simulink model "leader_qbot2"  (Simulink 8.3)
settings: Solver=ode1  StartTime=0.0  StopTime=inf  FixedStep=0.002  RelTol=1e-3
undefined symbols (not defined in the file or in its folder): HIL
libraries: quarc_library x13, simulink x1
settings Model: Creator=glai  LastModifiedBy=user  SimulationMode=external  ExtModeTrigDuration=5000
settings SolverCC: PositivePriorityOrder=on
settings DataIOCC: SignalLoggingSaveFormat=Dataset
settings OptimizationCC: ExpressionDepthLimit=2147483647
settings RTWCC: SystemTargetFile=quarc_linux_duovero.tlc  TemplateMakefile=quarc_linux_duovero_tmf  Description=QUARC Linux DuoVero Target (QBall 2, QBot 2)  ProcessScript=quarc_linux_duovero_make_rtw_hook
settings STFCustomTargetCC: TargetLibSuffix=.a  TargetPreCompLibLocation=C:\PROGRA~3\QUARC\lib\2014a\LINUX_~3\release  CodeReplacementLibrary=C89/C90 (ANSI)  ConcurrentExecutionCompliant=on  GeneratePreprocessorConditionals=Disable all  CombineOutputUpdateFcns=on  CPPClassGenCompliant=on  GRTInterface=off  SystemTargetFile=quarc_linux_duovero.tlc
settings GRTTargetCC: TargetLibSuffix=.a  TargetPreCompLibLocation=C:\PROGRA~3\QUARC\lib\2014a\LINUX_~3\release  CodeReplacementLibrary=C89/C90 (ANSI)  ParMdlRefBuildCompliant=off  CompOptLevelCompliant=off  CombineOutputUpdateFcns=on  MatFileLogging=off  GRTInterface=off  ExtMode=on  ExtModeMexFile=quarc_comm  ExtModeMexArgs='-w -d /tmp -uri %u', 'tcpip://192.168.2.47:17001?nagle=no,keep_alive=1'

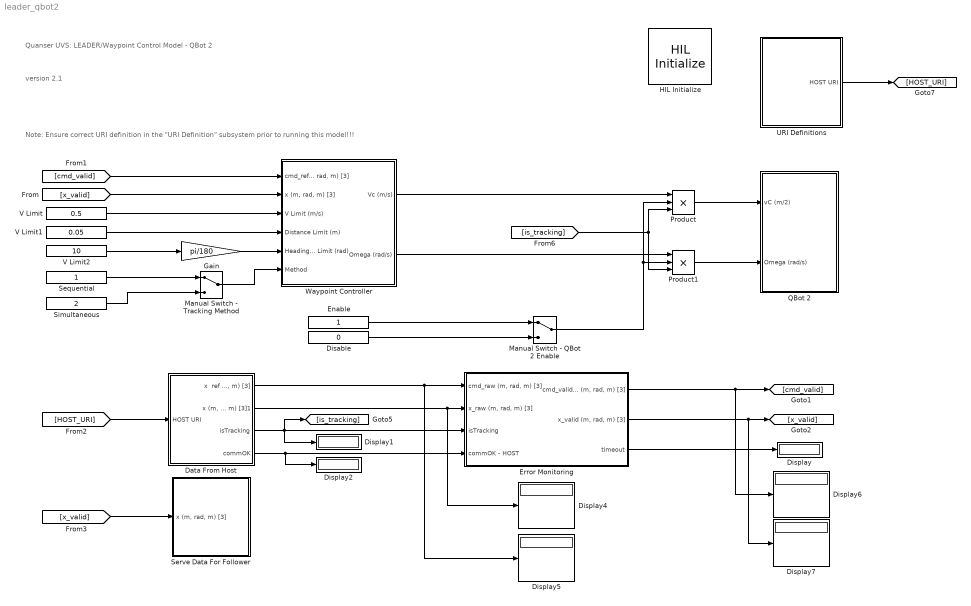
== system leader_qbot2 ==
  note: version 2.1
  note: Note: Ensure correct URI definition in the "URI Definition" subsystem prior to running this model!!!
  note: Quanser UVS: LEADER/Waypoint Control Model - QBot 2
  Data From Host : Subsystem
  Disable : Constant  Value=0
  Display{,1..2,4..7} (7 alike) : Display
      settings: Decimation=100
  Enable : Constant
  Error Monitoring : Subsystem
  Gain : Gain  Gain=pi/180
  HIL Initialize : quarc_library/Data Acquisition/Generic/Configuration/HIL Initialize  Priority=-99  object_name=HIL-1  board_type=qbot2  board_number=0  board_options=enc0_dir=0;enc0_filter=1;enc0_a=0;enc0_b=0;enc0_z=1;enc0_reload=0;enc1_dir=0;enc1_filter=1;enc1_a=0;enc1_b=0;enc1_z=1;enc1_reload=0;pwm0_immediate=0;pwm1_immediate=0;pwm2_immediate=0;pwm3_immediate=0;  exclusive=off  active=off  hardware_clocks=[]  clock_modes=[]  initial_clock_frequencies=[]  set_clock_params_at_start=off  set_clock_params_at_switch_in=off  set_clock_frequencies_at_start=off  set_clock_frequencies_at_switch_in=off  analog_input_channels=[0:9]  analog_input_maximums=[5 5 5 5 16.5 3.3 3.3 3.3 3.3]  analog_input_minimums=[0 0 0 0 0 0 0 0 0]  set_analog_input_params_at_start=off  set_analog_input_params_at_switch_in=off  analog_output_channels=[]  analog_output_maximums=[]  analog_output_minimums=[]  initial_analog_outputs=[]  final_analog_outputs=[]  watchdog_analog_outputs=[]  set_analog_output_params_at_start=off  set_analog_output_params_at_switch_in=off  set_analog_outputs_at_start=off  set_analog_outputs_at_switch_in=off  set_analog_outputs_at_terminate=off  set_analog_outputs_at_switch_out=off  set_analog_outputs_on_watchdog=off  digital_input_channels=[]  digital_output_channels=[]  digital_output_configuration=[]  initial_digital_outputs=[0]  final_digital_outputs=[0]  watchdog_digital_outputs=[0]  set_digital_output_params_at_start=off  set_digital_output_params_at_switch_in=off  set_digital_outputs_at_start=on  set_digital_outputs_at_switch_in=off  set_digital_outputs_at_terminate=on  set_digital_outputs_at_switch_out=off  set_digital_outputs_on_watchdog=on  encoder_channels=[0:3]  quadrature=[4]  encoder_filter_frequency=[]  initial_encoder_counts=[0]  set_encoder_params_at_start=on  set_encoder_params_at_switch_in=off  set_encoder_counts_at_start=on  set_encoder_counts_at_switch_in=off  pwm_channels=[0:3]  pwm_modes=[0]  pwm_frequency=[20e6/1024]  pwm_configuration=[0]  pwm_alignment=[0]  pwm_polarity=[1]  pwm_leading_deadband=[0]  pwm_trailing_deadband=[0]  initial_pwm_outputs=[0]  final_pwm_outputs=[0]  watchdog_pwm_outputs=[0]  set_pwm_params_at_start=on  set_pwm_params_at_switch_in=off  set_pwm_outputs_at_start=on  set_pwm_outputs_at_switch_in=off  set_pwm_outputs_at_terminate=on  set_pwm_outputs_at_switch_out=off  set_pwm_outputs_on_watchdog=on  other_output_channels=[2000:2001 14000 16000]  initial_other_outputs=[0 0 0 7]  final_other_outputs=[0 0 0 7]  watchdog_other_outputs=[]  set_other_outputs_at_start=on  set_other_outputs_at_switch_in=off  set_other_outputs_at_terminate=on  set_other_outputs_at_switch_out=off  set_other_outputs_on_watchdog=off
  Manual Switch - QBot 2 Enable : ManualSwitch
  Manual Switch - Tracking Method : ManualSwitch
  Product : Product  Inputs=3  RndMeth=Zero
  Product1 : Product  Inputs=3  RndMeth=Zero
  QBot 2 : Subsystem
  Sequential : Constant
  Serve Data For Follower : Subsystem
  Simultaneous : Constant  Value=2
  URI Definitions : Subsystem
  V Limit : Constant  Value=0.5
  V Limit1 : Constant  Value=0.05
  V Limit2 : Constant  Value=10
  Waypoint Controller : Subsystem
  wires:
  URI Definitions/1(HOST URI) -> [HOST_URI]
  [HOST_URI] -> Data From Host/1(HOST URI)
  Data From Host/3(isTracking) -> Error Monitoring/3(isTracking), Display1/1, [is_tracking]
  Data From Host/4(commOK) -> Display2/1, Error Monitoring/4(commOK - HOST)
  Error Monitoring/2("x_valid (m, rad, m) [3]") -> Display7/1, [x_valid]
  [x_valid] -> Waypoint Controller/2("x (m, rad, m) [3]")
  [cmd_valid] -> Waypoint Controller/1("cmd_ref (m, rad, m) [3]")
  V Limit1/1 -> Waypoint Controller/4(Distance Limit (m))
  V Limit/1 -> Waypoint Controller/3(V Limit (m/s))
  V Limit2/1 -> Gain/1
  Gain/1 -> Waypoint Controller/5(Heading Limit (rad))
  Sequential/1 -> Manual Switch - Tracking Method/1
  Simultaneous/1 -> Manual Switch - Tracking Method/2
  Manual Switch - Tracking Method/1 -> Waypoint Controller/6(Method)
  Enable/1 -> Manual Switch - QBot 2 Enable/1
  Disable/1 -> Manual Switch - QBot 2 Enable/2
  Waypoint Controller/1(Vc (m/s)) -> Product/1
  Product/1 -> QBot 2/1(vC (m/2))
  Waypoint Controller/2(Omega (rad/s)) -> Product1/1
  Product1/1 -> QBot 2/2(Omega (rad/s))
  Manual Switch - QBot 2 Enable/1 -> Product/2, Product1/2
  Error Monitoring/3(timeout) -> Display/1
  Error Monitoring/1("cmd_valid (m, rad, m) [3]") -> Display6/1, [cmd_valid]
  [is_tracking] -> Product1/3, Product/3
  Data From Host/1("x  ref (m, rad, m) [3]") -> Display5/1, Error Monitoring/1("cmd_raw (m, rad, m) [3]")
  Data From Host/2("x (m, rad, m) [3]1") -> Display4/1, Error Monitoring/2("x_raw (m, rad, m) [3]")
  [x_valid] -> Serve Data For Follower/1("x (m, rad, m) [3]")

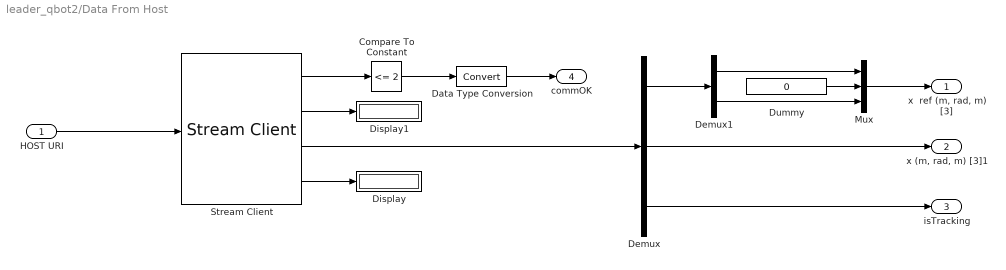
== system leader_qbot2/Data From Host ==
  HOST URI : Inport
  Compare To Constant : simulink/Logic and Bit Operations/Compare To Constant  relop=<=  const=2  OutDataTypeStr=boolean
  Data Type Conversion : DataTypeConversion
  Demux : Demux  Outputs=[2 3 1]
  Demux1 : Demux  Outputs=2
  Display : Display
      settings: Decimation=100
  Display1 : Display
      settings: Decimation=100
  Dummy : Constant  Value=0
  Mux : Mux  Inputs=3
  Stream Client : quarc_library/Communications/Basic/Stream Client  uri_source=External input port  uri=tcpip://182.168.2.222:18006  apply_uri_to_all_configs=on  send_buffer_size=1460  receive_buffer_size=1460  byte_order=little endian (Intel - LSB first)  optimization=Minimum latency  implementation=Use non-blocking I/O  send_options=Do not send data  receive_options=Receive most recent data  send_fifo_size=1000  receive_fifo_size=1000  send_priority=0  receive_priority=0  default_value=zeros(6,1)  send_dimensions=off  receive_dimensions=off  max_dimensions=-1  sample_time=qc_get_step_size  active=off  data_type=Inherited via back propagation  type_expr=BusObject
  "x  ref (m, rad, m) [3]" : Outport
  "x (m, rad, m) [3]1" : Outport  Port=2
  isTracking : Outport  Port=3
  commOK : Outport  Port=4
  wires:
  HOST URI/1 -> Stream Client/1
  Stream Client/2 -> Display1/1
  Stream Client/3 -> Demux/1
  Compare To Constant/1 -> Data Type Conversion/1
  Data Type Conversion/1 -> commOK/1
  Stream Client/1 -> Compare To Constant/1
  Stream Client/4 -> Display/1
  Demux/3 -> isTracking/1
  Demux/2 -> "x (m, rad, m) [3]1"/1
  Demux1/1 -> Mux/1
  Dummy/1 -> Mux/2
  Demux1/2 -> Mux/3
  Demux/1 -> Demux1/1
  Mux/1 -> "x  ref (m, rad, m) [3]"/1

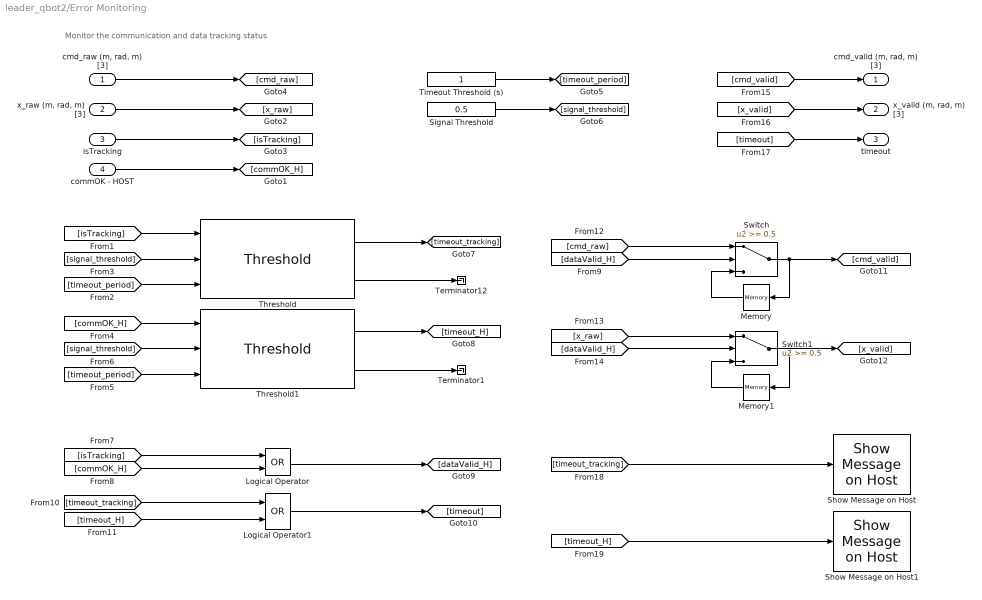
== system leader_qbot2/Error Monitoring ==
  note: Monitor the communication and data tracking status
  "cmd_raw (m, rad, m) [3]" : Inport
  "x_raw (m, rad, m) [3]" : Inport  Port=2
  isTracking : Inport  Port=3
  commOK - HOST : Inport  Port=4
  Logical Operator : Logic  Operator=OR  AllPortsSameDT=off  OutDataTypeStr=boolean
  Logical Operator1 : Logic  Operator=OR  AllPortsSameDT=off  OutDataTypeStr=boolean
  Memory : Memory
  Memory1 : Memory
  Show Message on Host : quarc_library/Sinks/Error Handling/Show Message on Host  message_type=Fixed error message  message_icon=Warning  message=OptiTrack Not Tracking Markers!
      settings: AttributesFormatString="\"%<message>\""
  Show Message on Host1 : quarc_library/Sinks/Error Handling/Show Message on Host  message_type=Fixed error message  message_icon=Warning  message=Host connection timeout detected!
      settings: AttributesFormatString="\"%<message>\""
  Signal Threshold : Constant  Value=0.5
  Switch : Switch  Threshold=0.5
  Switch1 : Switch  Threshold=0.5
  Terminator1 : Terminator
  Terminator12 : Terminator
  Threshold : quarc_library/Discontinuities/Threshold  operator=<  param_src=External input port  threshold=0  duration=0
  Threshold1 : quarc_library/Discontinuities/Threshold  operator=<  param_src=External input port  threshold=0  duration=0
  Timeout Threshold (s) : Constant
  "cmd_valid (m, rad, m) [3]" : Outport
  "x_valid (m, rad, m) [3]" : Outport  Port=2
  timeout : Outport  Port=3
  wires:
  "cmd_raw (m, rad, m) [3]"/1 -> [cmd_raw]
  "x_raw (m, rad, m) [3]"/1 -> [x_raw]
  isTracking/1 -> [isTracking]
  commOK - HOST/1 -> [commOK_H]
  Timeout Threshold (s)/1 -> [timeout_period]
  Signal Threshold/1 -> [signal_threshold]
  [timeout_period] -> Threshold/3
  [isTracking] -> Threshold/1
  [signal_threshold] -> Threshold/2
  [signal_threshold] -> Threshold1/2
  [timeout_period] -> Threshold1/3
  [commOK_H] -> Threshold1/1
  Threshold/1 -> [timeout_tracking]
  Threshold/2 -> Terminator12/1
  Threshold1/1 -> [timeout_H]
  Threshold1/2 -> Terminator1/1
  [commOK_H] -> Logical Operator/2
  [isTracking] -> Logical Operator/1
  Logical Operator/1 -> [dataValid_H]
  [timeout_H] -> Logical Operator1/2
  [timeout_tracking] -> Logical Operator1/1
  Logical Operator1/1 -> [timeout]
  [dataValid_H] -> Switch/2
  [cmd_raw] -> Switch/1
  Memory/1 -> Switch/3
  Switch/1 -> [cmd_valid], Memory/1
  [dataValid_H] -> Switch1/2
  [x_raw] -> Switch1/1
  Memory1/1 -> Switch1/3
  Switch1/1 -> [x_valid], Memory1/1
  [cmd_valid] -> "cmd_valid (m, rad, m) [3]"/1
  [x_valid] -> "x_valid (m, rad, m) [3]"/1
  [timeout] -> timeout/1
  [timeout_tracking] -> Show Message on Host/1
  [timeout_H] -> Show Message on Host1/1

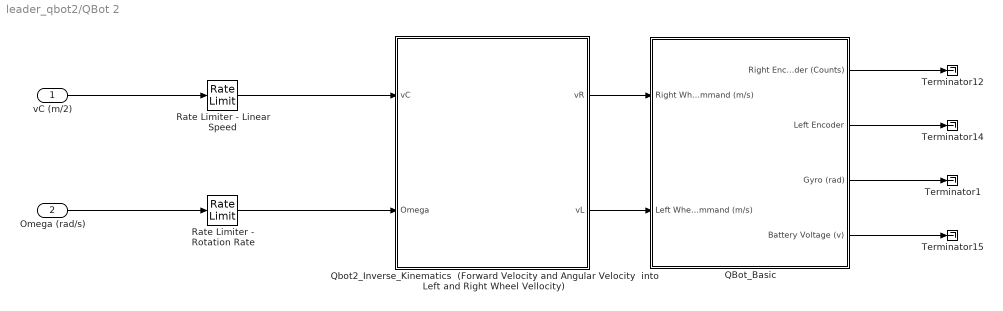
== system leader_qbot2/QBot 2 ==
  vC (m/2) : Inport
  Omega (rad/s) : Inport  Port=2
  QBot_Basic : Subsystem
  Qbot2_Inverse_Kinematics  (Forward Velocity and Angular Velocity  into Left and Right Wheel Vellocity) : Subsystem
  Rate Limiter - Linear Speed : RateLimiter  SampleTimeMode=inherited
  Rate Limiter - Rotation Rate : RateLimiter  SampleTimeMode=inherited
  Terminator{1,12,14..15} (4 alike) : Terminator
  wires:
  Qbot2_Inverse_Kinematics  (Forward Velocity and Angular Velocity  into Left and Right Wheel Vellocity)/1(vR) -> QBot_Basic/1(Right Wheel Command (m/s))
  Qbot2_Inverse_Kinematics  (Forward Velocity and Angular Velocity  into Left and Right Wheel Vellocity)/2(vL) -> QBot_Basic/2(Left Wheel Command (m/s))
  QBot_Basic/1(Right Encoder (Counts)) -> Terminator12/1
  QBot_Basic/4(Battery Voltage (v)) -> Terminator15/1
  QBot_Basic/2(Left Encoder) -> Terminator14/1
  vC (m/2)/1 -> Rate Limiter - Linear Speed/1
  Omega (rad/s)/1 -> Rate Limiter - Rotation Rate/1
  QBot_Basic/3(Gyro (rad)) -> Terminator1/1
  Rate Limiter - Linear Speed/1 -> Qbot2_Inverse_Kinematics  (Forward Velocity and Angular Velocity  into Left and Right Wheel Vellocity)/1(vC)
  Rate Limiter - Rotation Rate/1 -> Qbot2_Inverse_Kinematics  (Forward Velocity and Angular Velocity  into Left and Right Wheel Vellocity)/2(Omega)

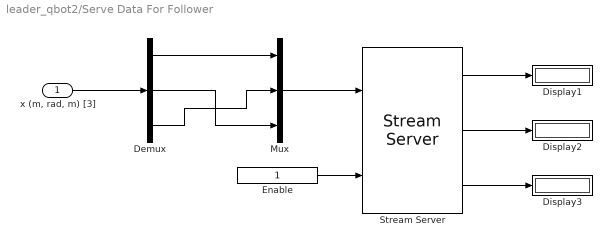
== system leader_qbot2/Serve Data For Follower ==
  "x (m, rad, m) [3]" : Inport
  Demux : Demux  Outputs=3
  Display1 : Display
      settings: Decimation=100
  Display2 : Display
      settings: Decimation=100
  Display3 : Display
      settings: Decimation=100
  Enable : Constant
  Mux : Mux  Inputs=3
  Stream Server : quarc_library/Communications/Basic/Stream Server  uri_source=Specify via dialog (do not evaluate)  uri=tcpip://localhost:18007  apply_uri_to_all_configs=on  send_buffer_size=1460  receive_buffer_size=1460  byte_order=little endian (Intel - LSB first)  optimization=Minimum latency  implementation=Use non-blocking I/O  send_options=Send most recent data  receive_options=Do not receive data  send_fifo_size=1000  receive_fifo_size=1000  send_priority=0  receive_priority=0  default_value=[0]  send_dimensions=off  receive_dimensions=off  max_dimensions=-1  sample_time=qc_get_step_size  active=off  data_type=Inherited via back propagation  type_expr=BusObject
      settings: AttributesFormatString="\"tcpip://localhost:18007\""
  wires:
  Mux/1 -> Stream Server/1
  Enable/1 -> Stream Server/2
  Stream Server/3 -> Display3/1
  Stream Server/2 -> Display2/1
  Stream Server/1 -> Display1/1
  Demux/1 -> Mux/1
  Demux/2 -> Mux/3
  Demux/3 -> Mux/2
  "x (m, rad, m) [3]"/1 -> Demux/1

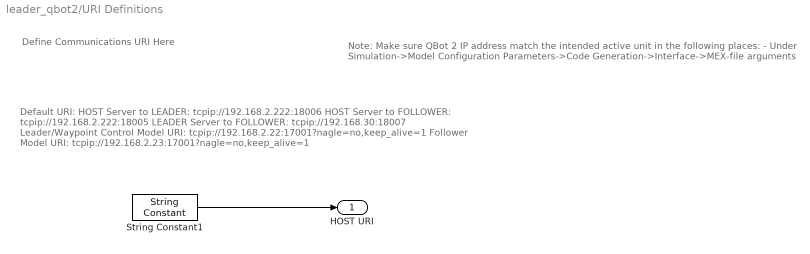
== system leader_qbot2/URI Definitions ==
  note: Note: Make sure QBot 2 IP address match the intended active unit in the following places:
      | - Under Simulation->Model Configuration Parameters->Code Generation->Interface->MEX-file arguments
  note: Default URI:
      |
      | HOST Server to LEADER: tcpip://192.168.2.222:18006
      | HOST Server to FOLLOWER: tcpip://192.168.2.222:18005
      | LEADER Server to FOLLOWER: tcpip://192.168.30:18007
      |
      | Leader/Waypoint Control Model URI: tcpip://192.168.2.22:17001?nagle=no,keep_alive=1
      | Follower Model URI: tcpip://192.168.2.23:17001?nagle=no,keep_alive=1
  note: Define Communications URI Here
  String Constant1 : quarc_library/Strings/String Constant  string_value=tcpip://192.168.2.10:18006  evaluate_string=off  string_type=text  max_length=80  sample_time=inf  variable_size=off
      settings: AttributesFormatString="\"tcpip://192.168.2.10:18006\""
  HOST URI : Outport
  wires:
  String Constant1/1 -> HOST URI/1

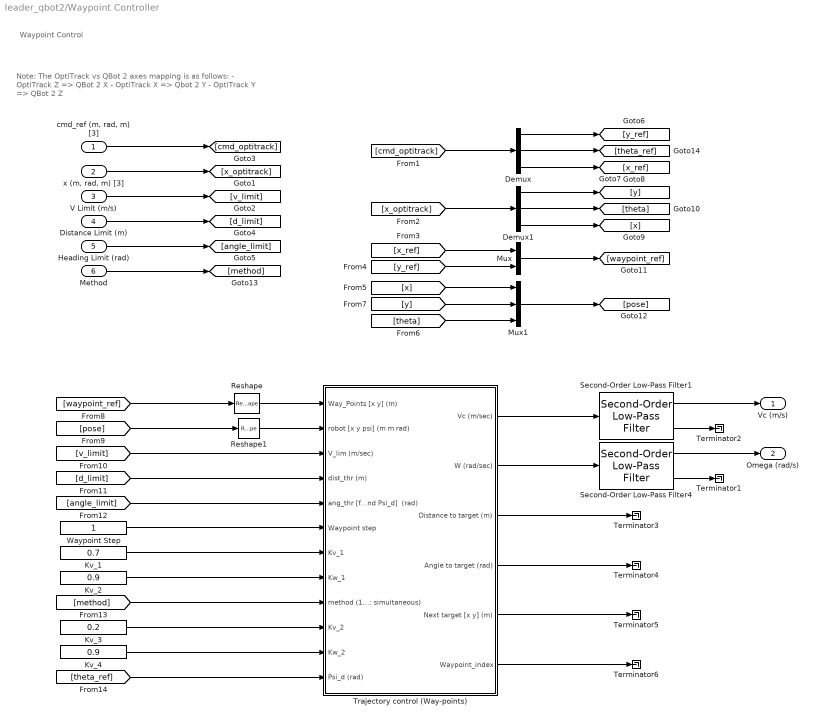
== system leader_qbot2/Waypoint Controller ==
  note: Note: The OptiTrack vs QBot 2 axes mapping is as follows:
      |
      | - OptiTrack Z => QBot 2 X
      | - OptiTrack X => Qbot 2 Y
      | - OptiTrack Y => QBot 2 Z
  note: Waypoint Control
  "cmd_ref (m, rad, m) [3]" : Inport
  "x (m, rad, m) [3]" : Inport  Port=2
  V Limit (m/s) : Inport  Port=3
  Distance Limit (m) : Inport  Port=4
  Heading Limit (rad) : Inport  Port=5
  Method : Inport  Port=6
  Demux : Demux  Outputs=3
  Demux1 : Demux  Outputs=3
  Kv_1 : Constant  Value=0.7
  Kv_2 : Constant  Value=0.9
  Kv_3 : Constant  Value=0.2
  Kv_4 : Constant  Value=0.9
  Mux : Mux  Inputs=2
  Mux1 : Mux  Inputs=3
  Reshape : Reshape  OutputDimensionality=Row vector (2-D)
  Reshape1 : Reshape  OutputDimensionality=Column vector (2-D)
  Second-Order Low-Pass Filter1 : quarc_library/Continuous/Second-Order Low-Pass Filter  params_source=Internal (dialog parameters)  input_width=30  input_zeta=1  input_init=0
  Second-Order Low-Pass Filter4 : quarc_library/Continuous/Second-Order Low-Pass Filter  params_source=Internal (dialog parameters)  input_width=60  input_zeta=1  input_init=0
  Terminator{1..6} (6 alike) : Terminator
  Trajectory control (Way-points) : Subsystem
  Waypoint Step : Constant
  Vc (m/s) : Outport
  Omega (rad/s) : Outport  Port=2
  wires:
  "cmd_ref (m, rad, m) [3]"/1 -> [cmd_optitrack]
  "x (m, rad, m) [3]"/1 -> [x_optitrack]
  V Limit (m/s)/1 -> [v_limit]
  Distance Limit (m)/1 -> [d_limit]
  Heading Limit (rad)/1 -> [angle_limit]
  Demux/3 -> [x_ref]
  Demux/1 -> [y_ref]
  [cmd_optitrack] -> Demux/1
  Demux1/3 -> [x]
  Demux1/1 -> [y]
  [x_optitrack] -> Demux1/1
  Demux1/2 -> [theta]
  [x_ref] -> Mux/1
  [y_ref] -> Mux/2
  Mux/1 -> [waypoint_ref]
  Mux1/1 -> [pose]
  [x] -> Mux1/1
  [waypoint_ref] -> Reshape/1
  Reshape/1 -> Trajectory control (Way-points)/1(Way_Points [x y] (m))
  [pose] -> Reshape1/1
  Reshape1/1 -> Trajectory control (Way-points)/2(robot [x y psi] (m m rad))
  Trajectory control (Way-points)/1(Vc (m/sec)) -> Second-Order Low-Pass Filter1/1
  Trajectory control (Way-points)/2(W (rad/sec)) -> Second-Order Low-Pass Filter4/1
  Second-Order Low-Pass Filter1/1 -> Vc (m/s)/1
  Second-Order Low-Pass Filter1/2 -> Terminator2/1
  Second-Order Low-Pass Filter4/1 -> Omega (rad/s)/1
  Second-Order Low-Pass Filter4/2 -> Terminator1/1
  [v_limit] -> Trajectory control (Way-points)/3(V_lim (m/sec))
  [d_limit] -> Trajectory control (Way-points)/4(dist_thr (m))
  [angle_limit] -> Trajectory control (Way-points)/5(ang_thr [for method 1 and Psi_d]  (rad))
  Waypoint Step/1 -> Trajectory control (Way-points)/6(Waypoint step)
  Kv_1/1 -> Trajectory control (Way-points)/7(Kv_1)
  Kv_2/1 -> Trajectory control (Way-points)/8(Kw_1)
  Method/1 -> [method]
  [method] -> Trajectory control (Way-points)/9("method (1: sequential, 2: simultaneous)")
  Kv_3/1 -> Trajectory control (Way-points)/10(Kv_2)
  Kv_4/1 -> Trajectory control (Way-points)/11(Kw_2)
  [theta_ref] -> Trajectory control (Way-points)/12(Psi_d (rad))
  Demux/2 -> [theta_ref]
  Trajectory control (Way-points)/6(Waypoint_index) -> Terminator6/1
  Trajectory control (Way-points)/5(Next target [x y] (m)) -> Terminator5/1
  Trajectory control (Way-points)/4(Angle to target (rad)) -> Terminator4/1
  Trajectory control (Way-points)/3(Distance to target (m)) -> Terminator3/1
  [y] -> Mux1/2
  [theta] -> Mux1/3

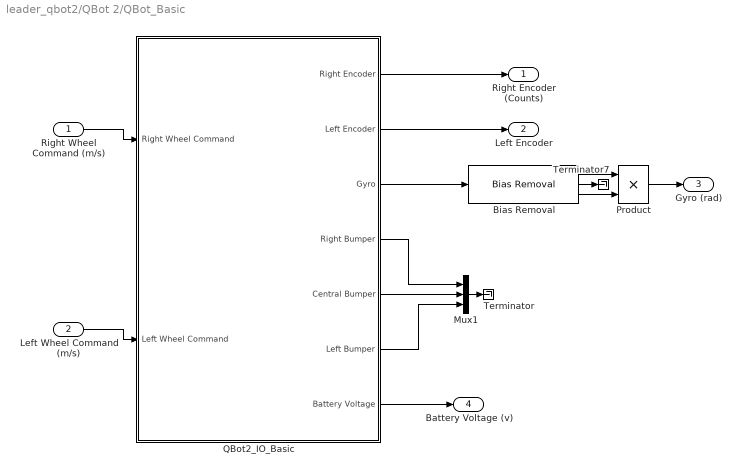
== system leader_qbot2/QBot 2/QBot_Basic ==
  Right Wheel Command (m/s) : Inport
  Left Wheel Command (m/s) : Inport  Port=2
  Bias Removal : quarc_library/Discrete/Bias Removal  start_time=3  end_time=4  switch_id=0  sample_time=qc_get_step_size
  Mux1 : Mux  Inputs=3
  Product : Product  RndMeth=Zero
  QBot2_IO_Basic : Subsystem
  Terminator : Terminator
  Terminator7 : Terminator
  Right Encoder (Counts) : Outport
  Left Encoder : Outport  Port=2
  Gyro (rad) : Outport  Port=3
  Battery Voltage (v) : Outport  Port=4
  wires:
  QBot2_IO_Basic/4(Right Bumper) -> Mux1/1
  QBot2_IO_Basic/5(Central Bumper) -> Mux1/2
  QBot2_IO_Basic/6(Left Bumper) -> Mux1/3
  Right Wheel Command (m/s)/1 -> QBot2_IO_Basic/1(Right Wheel Command)
  Left Wheel Command (m/s)/1 -> QBot2_IO_Basic/2(Left Wheel Command)
  QBot2_IO_Basic/1(Right Encoder) -> Right Encoder (Counts)/1
  QBot2_IO_Basic/2(Left Encoder) -> Left Encoder/1
  QBot2_IO_Basic/7(Battery Voltage) -> Battery Voltage (v)/1
  Bias Removal/2 -> Terminator7/1
  Bias Removal/1 -> Product/1
  Bias Removal/3 -> Product/2
  Product/1 -> Gyro (rad)/1
  QBot2_IO_Basic/3(Gyro) -> Bias Removal/1
  Mux1/1 -> Terminator/1

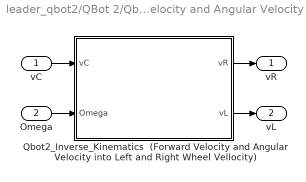
== system leader_qbot2/QBot 2/Qbot2_Inverse_Kinematics  (Forward Velocity and Angular Velocity  into Left and Right Wheel Vellocity) ==
  vC : Inport
  Omega : Inport  Port=2
  Qbot2_Inverse_Kinematics  (Forward Velocity and Angular Velocity into Left and Right Wheel Vellocity) : MATLAB Function  TreatAsAtomicUnit=on
  vR : Outport
  vL : Outport  Port=2
  wires:
  vC/1 -> Qbot2_Inverse_Kinematics  (Forward Velocity and Angular Velocity into Left and Right Wheel Vellocity)/1(vC)
  Qbot2_Inverse_Kinematics  (Forward Velocity and Angular Velocity into Left and Right Wheel Vellocity)/1(vR) -> vR/1
  Omega/1 -> Qbot2_Inverse_Kinematics  (Forward Velocity and Angular Velocity into Left and Right Wheel Vellocity)/2(Omega)
  Qbot2_Inverse_Kinematics  (Forward Velocity and Angular Velocity into Left and Right Wheel Vellocity)/2(vL) -> vL/1

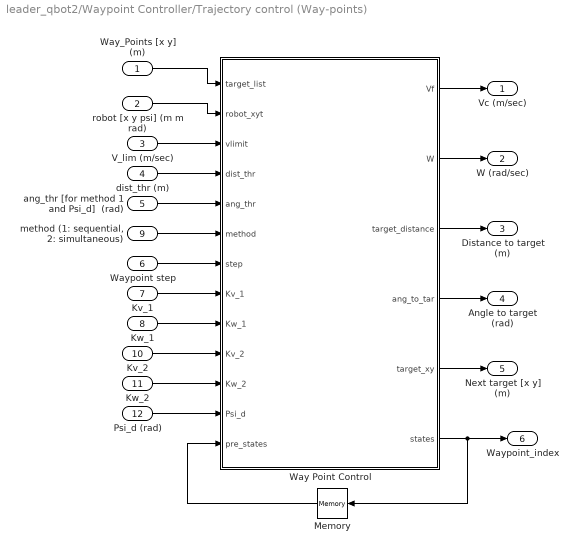
== system leader_qbot2/Waypoint Controller/Trajectory control (Way-points) ==
  Way_Points [x y] (m) : Inport
  robot [x y psi] (m m rad) : Inport  Port=2
  V_lim (m/sec) : Inport  Port=3
  dist_thr (m) : Inport  Port=4
  ang_thr [for method 1 and Psi_d]  (rad) : Inport  Port=5
  Waypoint step : Inport  Port=6
  Kv_1 : Inport  Port=7
  Kw_1 : Inport  Port=8
  "method (1: sequential, 2: simultaneous)" : Inport  Port=9
  Kv_2 : Inport  Port=10
  Kw_2 : Inport  Port=11
  Psi_d (rad) : Inport  Port=12
  Memory : Memory  X0=[0]
  Way Point Control : MATLAB Function  TreatAsAtomicUnit=on
  Vc (m/sec) : Outport
  W (rad/sec) : Outport  Port=2
  Distance to target (m) : Outport  Port=3
  Angle to target (rad) : Outport  Port=4
  Next target [x y] (m) : Outport  Port=5
  Waypoint_index : Outport  Port=6
  wires:
  Psi_d (rad)/1 -> Way Point Control/12(Psi_d)
  Kw_2/1 -> Way Point Control/11(Kw_2)
  Kv_2/1 -> Way Point Control/10(Kv_2)
  "method (1: sequential, 2: simultaneous)"/1 -> Way Point Control/6(method)
  Kw_1/1 -> Way Point Control/9(Kw_1)
  Way Point Control/5(target_xy) -> Next target [x y] (m)/1
  Kv_1/1 -> Way Point Control/8(Kv_1)
  Waypoint step/1 -> Way Point Control/7(step)
  Way Point Control/4(ang_to_tar) -> Angle to target (rad)/1
  ang_thr [for method 1 and Psi_d]  (rad)/1 -> Way Point Control/5(ang_thr)
  Way Point Control/3(target_distance) -> Distance to target (m)/1
  dist_thr (m)/1 -> Way Point Control/4(dist_thr)
  Way Point Control/2(W) -> W (rad/sec)/1
  V_lim (m/sec)/1 -> Way Point Control/3(vlimit)
  robot [x y psi] (m m rad)/1 -> Way Point Control/2(robot_xyt)
  Way Point Control/1(Vf) -> Vc (m/sec)/1
  Way_Points [x y] (m)/1 -> Way Point Control/1(target_list)
  Way Point Control/6(states) -> Waypoint_index/1, Memory/1
  Memory/1 -> Way Point Control/13(pre_states)

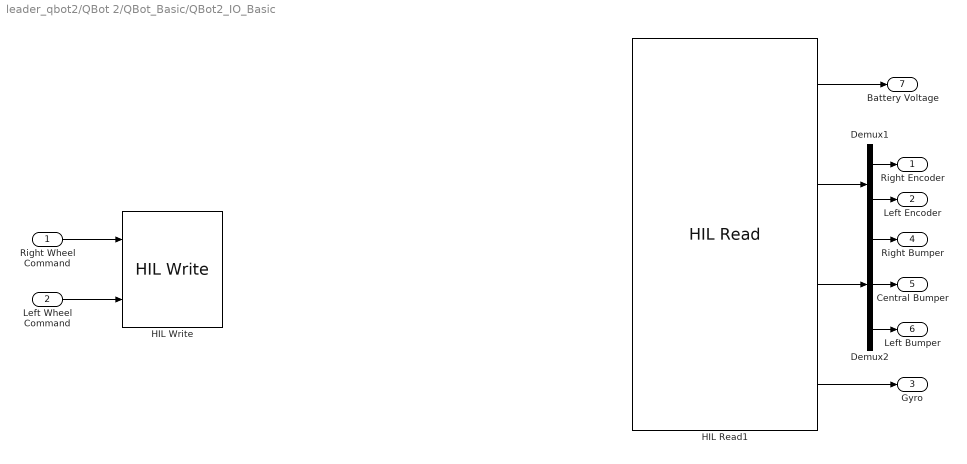
== system leader_qbot2/QBot 2/QBot_Basic/QBot2_IO_Basic ==
  Right Wheel Command : Inport
  Left Wheel Command : Inport  Port=2
  Demux1 : Demux  Outputs=2
  Demux2 : Demux  Outputs=3
  HIL Read1 : quarc_library/Data Acquisition/Generic/Immediate I//O/HIL Read  object_name=HIL-1  analog_channels=[4]  encoder_channels=[2 3]  digital_channels=[8 9 10]  other_channels=[1002]  sample_time=qc_get_step_size  active=on  vector_output=on  data_type_mode=Inherit via back propagation  encoder_data_type=double  digital_data_type=boolean
  HIL Write : quarc_library/Data Acquisition/Generic/Immediate I//O/HIL Write  object_name=HIL-1  analog_channels=[]  pwm_channels=[]  digital_channels=[]  other_channels=[2000:2001]  sample_time=-1  active=on  vector_input=off
  Right Encoder : Outport
  Left Encoder : Outport  Port=2
  Gyro : Outport  Port=3
  Right Bumper : Outport  Port=4
  Central Bumper : Outport  Port=5
  Left Bumper : Outport  Port=6
  Battery Voltage : Outport  Port=7
  wires:
  HIL Read1/1 -> Battery Voltage/1
  HIL Read1/3 -> Demux2/1
  HIL Read1/4 -> Gyro/1
  Demux1/1 -> Right Encoder/1
  Demux1/2 -> Left Encoder/1
  Right Wheel Command/1 -> HIL Write/1
  Left Wheel Command/1 -> HIL Write/2
  HIL Read1/2 -> Demux1/1
  Demux2/1 -> Right Bumper/1
  Demux2/2 -> Central Bumper/1
  Demux2/3 -> Left Bumper/1

== matlab function QBot 2/Qbot2_Inverse_Kinematics (Forward Velocity and Angular Velocity into Left and Right Wheel Vellocity)/Qbot2_Inverse_Kinematics (Forward Velocity and Angular Velocity into Left and Right Wheel Vellocity) ==
  data: vR output double; vL output double; vC input double; Omega input double
function [vR,vL] = fcn(vC , Omega)
%#codegen

d=0.235; 
% Eqn Based on the eqn 4.52 (W is the angular velocity)

vR = vC + Omega*d/2;
vL= vC - Omega*d/2;

== matlab function Waypoint Controller/Trajectory control (Way-points)/Way Point Control ==
  data: target_list input double; robot_xyt input double; vlimit input double; dist_thr input double; ang_thr input double; method input double; step input double; Kv_1 input double; Kw_1 input double; Kv_2 input double; Kw_2 input double; Psi_d input double; Vf output double; W output double; target_distance output double; ang_to_tar output double; target_xy output double; states output double; pre_states input double
function [Vf, W, target_distance, ang_to_tar, target_xy, states] = ...
    WaypointControl(target_list, robot_xyt, vlimit, ...
    dist_thr, ang_thr, method, step, Kv_1, Kw_1, Kv_2, Kw_2, Psi_d, pre_states)

% Initialize output variables

 Vf=0;
 W=0;
 finished_path_flag=0; 
 
 persistent Vf_1 end_flag;
 
 if isempty(Vf_1)
     Vf_1=0;
 end
 if isempty(end_flag)
    end_flag = 0;
 end
states = pre_states;



rx = robot_xyt(1);
ry = robot_xyt(2);
rtheta = check_angle(robot_xyt(3));
target_xy = [rx ry];
[n xy] = size(target_list);
if n==2 && xy==1
    target_xy = [target_list(1,1) target_list(2,1)];
    n = 1;
else
    for i=1:n
        if states(1) == i
            for j=1:xy
                target_xy(j) = target_list(i, j);
            end
        end
    end
end

tx = target_xy(1);
ty = target_xy(2);
target_distance = find_dist(rx, ry, tx, ty);
ang_to_tar= find_theta(rx, ry, rtheta, tx, ty);

if ((states(1) == n) && (target_distance <= dist_thr))  %|| states(1) == -1
% %        states(1) = -1;
       % right_vel = int16(0);
       % left_vel = int16(0);
%  %       target_distance = 0;
        Vf=0;
        W=0;
        
       if (end_flag == 1) && (target_distance <= dist_thr) % after all waypoints, psi will be adjusted to psi_d 
            [Vf, W] = ClosedLoop_Sequential(0, check_angle(check_angle(Psi_d)-check_angle(rtheta)), vlimit, ang_thr, dist_thr, Kv_1, Kw_1, Vf_1); 
             Vf_1=Vf;
       end
        
   
else
    
    if (target_distance <= dist_thr) && (end_flag==0)
            states(1) = pre_states(1) + step;%1;
    
     if (pre_states(1)>0)
         while (abs((target_list(states(1),1))-(target_list(pre_states(1),1)))<2*dist_thr) && (abs((target_list(states(1),2))-(target_list(pre_states(1),2)))<2*dist_thr)
             if (states(1)<=(n-step))
                 states(1) = states(1) + step;%1;
             else
                 states(1)=n;
             end
         end
     else 
          states(1) = states(1) + step;%1;
     end
          
         if states(1) >= n 
            states(1) = n;
            end_flag=1;
         end
        
               
  %  elseif (end_flag == 1) && (target_distance <= dist_thr) % after all waypoints, psi will be adjusted to psi_d 
  %          [Vf, W] = ClosedLoop_Sequential(0, check_angle(check_angle(Psi_d)-check_angle(rtheta)), vlimit, ang_thr, dist_thr, Kv_1, Kw_1, Vf_1); 
  %           Vf_1=Vf;
    else
        
        
            if method == 2
                [Vf, W] = ClosedLoop_Both(target_distance,  ang_to_tar, vlimit, Kv_2, Kw_2);    
            else
    %            [right_vel, left_vel] = rotate_and_go(ang_to_tar, vlimit, ang_thr);
                [Vf, W] = ClosedLoop_Sequential(target_distance,  ang_to_tar, vlimit, ang_thr, dist_thr, Kv_1, Kw_1, Vf_1); 
                Vf_1=Vf;
            end
                 
    end
end


return;

%--------------------------------------------------------------------------
function [y] = check_angle(x)
y = x;
if x > pi
    y = x - 2*pi;
elseif x < -pi
    y = x + 2*pi;
end
return;
% -------------------------------------------------------------------------
function dist = find_dist(rx, ry, tx, ty)
dist = sqrt((rx-tx)^2 + (ry-ty)^2);
return;
% -------------------------------------------------------------------------
function [theta]= find_theta(rx, ry, rtheta, tx, ty)

X = tx - rx;
Y = ty - ry;
theta = atan2(Y, X);
theta = check_angle(check_angle(theta)-check_angle(rtheta));

return;
% -------------------------------------------------------------------------

function [Vf, W] = ClosedLoop_Both(dist, theta, vlimit, Kv,Kw)

d = 0.23;
vmax = vlimit;
wmax = (2*vmax);
W = Kw*theta;

%if abs(theta)<pi
Vf = Kv*dist;
%else
%    Vf=0;
%end

w_sign = sign(W);
if abs(W) > wmax
    W = w_sign*wmax;
end
if abs(Vf)> vlimit
    Vf = abs(Vf)*vlimit;
end

return;

function [Vf, W] = ClosedLoop_Sequential(dist, theta, vlimit, ang_thr, dist_thr, Kv, Kw, Vf_1)

d = 0.23;
vmax = vlimit;
wmax = (2*vmax);

if (((abs(theta) > ang_thr))  && (Vf_1<0.01)) || (abs(theta) > 5*ang_thr) % once rotated, then moves. once started moving, it won't turn unless the heading is too off target or have reached the previous target.
        W=Kw*theta;
        Vf=0;
        if abs(W)> wmax
            W=sign(theta)*wmax;
        end
else
        Vf=Kv*dist;
       
        if abs(Vf)>vlimit
            Vf=sign(Vf)*vlimit;
        end
       % if (abs(theta) > 2*ang_thr)
       %   W=Kw*theta;
       %   Vf=0.4*Vf;
       % else
       W=0;
       % end
       % if abs(W)> wmax
       %     W=sign(theta)*wmax;
       % end
        
end

return;

%{
function [vr, vl] = solve_inv_kin(dist, theta, vlimit, delta_t)

d = 0.23;
vmax = vlimit(2);
wmax = (2*vmax)/d;
w = theta/delta_t;
w_sign = sign(w);
if abs(w) > wmax
    w = w_sign*wmax;
    vr = int16(round((d*w)/2));
    vl = int16(-vr);
else
    v = dist/delta_t;
    vr_tmp = (2*v + d*w)/2;
    vl_tmp = 2*v - vr_tmp;
    
    max_of_vrvl = abs(max(vr_tmp, vl_tmp));
    if max_of_vrvl > vmax
        vr_tmp = (vr_tmp/max_of_vrvl)*vmax;
        vl_tmp = (vl_tmp/max_of_vrvl)*vmax;
    end
    vr = int16(vr_tmp);
    vl = int16(vl_tmp);

end


return;
%}

%{
% -------------------------------------------------------------------------
function [vr, vl] = rotate_and_go(theta, vlimit, ang_thr)

if abs(theta) > ang_thr
    if theta >= 0
        vr = int16(vlimit(1));
        vl = int16(-vlimit(1));
    else
        vr = int16(-vlimit(1));
        vl = int16(vlimit(1));
    end
else
        vr = int16(vlimit(2));
        vl = int16(vlimit(2));
end

return;
% -------------------------------------------------------------------------
%}
